simulink model "Dcmodel"  (Simulink 7.9)
settings: Solver=ode45  StartTime=0.0  StopTime=10.0  RelTol=1e-3
undefined symbols (not defined in the file): B, J, kb, La, Ra, Tl, Vs
settings Model: Creator=PG  LastModifiedBy=PG

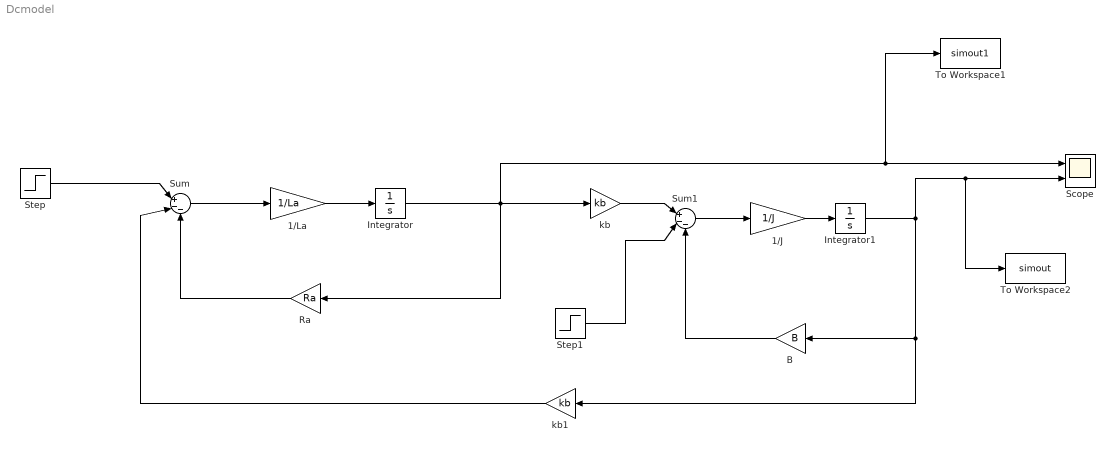
== system Dcmodel ==
  1/J : Gain  Gain=1/J
  1/La : Gain  Gain=1/La
  B : Gain  Gain=B
  Integrator : Integrator
  Integrator1 : Integrator
  Ra : Gain  Gain=Ra
  Scope : Scope  NumInputPorts=2
      settings: YMin=-5~-5  YMax=5~5
  Step : Step  After=Vs  SampleTime=0
  Step1 : Step  Time=2  After=Tl  SampleTime=0
  Sum : Sum  Inputs=|+--
  Sum1 : Sum  Inputs=|+--
  To Workspace1 : ToWorkspace  VariableName=simout1  SampleTime=-1  SaveFormat=Timeseries
  To Workspace2 : ToWorkspace  VariableName=simout  SampleTime=-1  SaveFormat=Timeseries
  kb : Gain  Gain=kb
  kb1 : Gain  Gain=kb
  wires:
  1/La/1 -> Integrator/1
  Sum/1 -> 1/La/1
  Integrator/1 -> Ra/1, kb/1, Scope/1, To Workspace1/1
  Step/1 -> Sum/1
  Ra/1 -> Sum/3
  kb/1 -> Sum1/1
  Step1/1 -> Sum1/2
  Sum1/1 -> 1/J/1
  1/J/1 -> Integrator1/1
  Integrator1/1 -> B/1, kb1/1, Scope/2, To Workspace2/1
  B/1 -> Sum1/3
  kb1/1 -> Sum/2
